simulink model "observateur_terme_integral"  (R2025b)
settings: Solver=FixedStepAuto  StartTime=0.0  StopTime=inf  RelTol=1e-3  EnableMultiTasking=on
values from neighbouring files (symbols this model uses):
  H_barre = K_t(3)    [AncienTest.m]
  K_int = K_t(1:2)    [AncienTest.m]
  Te = 1/100    (= 0.01)    [AncienTest.m]    (also in Test.m)
undefined symbols (not defined in the file or in its folder): Aobs, Bobs, Cobs, Dobs
libraries: legoev3lib x2
settings Model: ExtModeTrigDuration=2  Creator=carol  LastModifiedBy=carol
settings SolverCC: PositivePriorityOrder=on
settings OptimizationCC: DefaultParameterBehavior=Inlined  EnhancedBackFolding=on  PassReuseOutputArgsAs=Individual arguments  ZeroExternalMemoryAtStartup=off  ZeroInternalMemoryAtStartup=off  MaxStackSize=64  OptimizeBlockOrder=speed  DifferentSizesBufferReuse=on  OptimizationCustomize=off  EfficientTunableParamExpr=on
settings DebuggingCC: ParameterTunabilityLossMsg=error
settings HardwareCC: ProdBitPerPointer=32.0  ProdBitPerSizeT=32.0  ProdBitPerPtrDiffT=32.0  ProdLargestAtomicInteger=Long  ProdWordSize=32.0  ProdHWDeviceType=ARM Compatible->ARM 9  UseEmbeddedCoderFeatures=off  UseSimulinkCoderFeatures=off
settings SFSimCC: MATLABDynamicMemAlloc=off
settings RTWCC: SystemTargetFile=ert.tlc  HardwareBoard=LEGO MINDSTORMS EV3  TLCOptions="-aInlineSetEventsForThisBaseRateFcn=TLC_FALSE -aSuppressMultiTaskScheduler=TLC_FALSE  -aRateBasedStepFcn=0"  TemplateMakefile=ert_default_tmf  Toolchain=Sourcery G++ Lite v2009q3  Description=Embedded Coder
settings CodeAppCC: ForceParamTrailComments=on  IgnoreCustomStorageClasses=off  OperatorAnnotations=on  SimulinkDataObjDesc=on  SFDataObjDesc=on  InsertBlockDesc=on
settings ERTTargetCC: ExtModeTransport=2.0  ExtModeStaticAlloc=on  ExtModeMexFile=ext_xcp  ExtModeIntrfLevel=Level2 - Open  SupportContinuousTime=on  SupportNonInlinedSFcns=on  SupportVariableSizeSignals=on

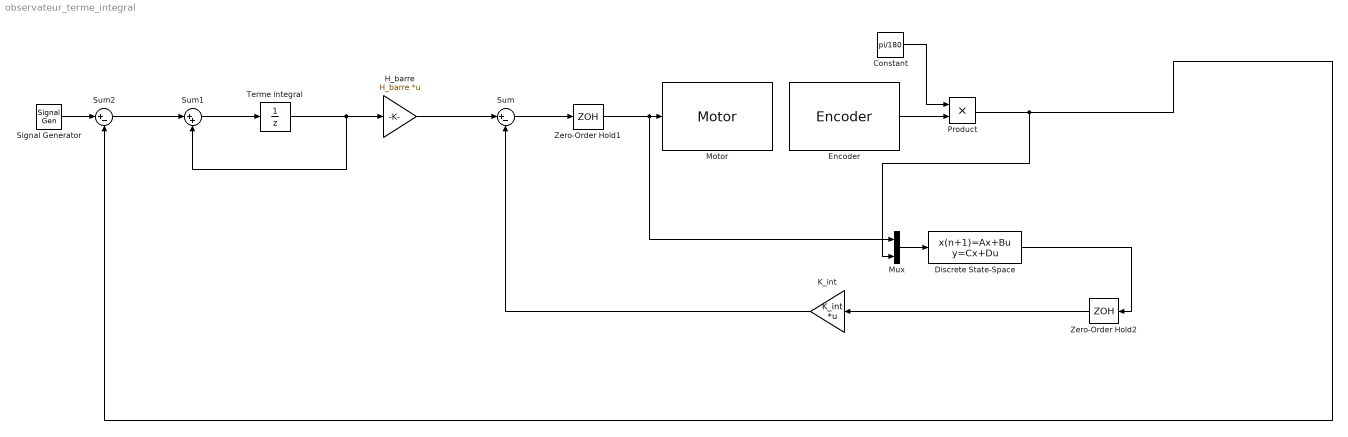
== system observateur_terme_integral ==
  Constant : Constant  Value=pi/180
  Discrete State-Space : DiscreteStateSpace  A=Aobs  B=Bobs  C=Cobs  D=Dobs  SampleTime=Te
  Encoder : legoev3lib/Encoder  portNumber=D  opMode=Reset by external signal  sampleTime=Te
  H_barre : Gain  Gain=H_barre  Multiplication=Matrix(K*u)
  K_int : Gain  Gain=K_int  Multiplication=Matrix(K*u)
  Motor : legoev3lib/Motor  sportNumber=D  sstopAction=Brake
  Mux : Mux  Inputs=2
  Product : Product
  Signal Generator : SignalGenerator  WaveForm=square  Frequency=0.1
  Sum : Sum  Inputs=|+-
  Sum1 : Sum  Inputs=|++
  Sum2 : Sum  Inputs=|+-
  Terme integral : UnitDelay  SampleTime=-1  HasFrameUpgradeWarning=on
  Zero-Order Hold1 : ZeroOrderHold  SampleTime=Te
  Zero-Order Hold2 : ZeroOrderHold  SampleTime=Te
  wires:
  Encoder/1 -> Product/2
  Zero-Order Hold1/1 -> Mux/1, Motor/1
  Sum/1 -> Zero-Order Hold1/1
  H_barre/1 -> Sum/1
  K_int/1 -> Sum/2
  Product/1 -> Mux/2, Sum2/2
  Constant/1 -> Product/1
  Zero-Order Hold2/1 -> K_int/1
  Terme integral/1 -> Sum1/2, H_barre/1
  Sum1/1 -> Terme integral/1
  Sum2/1 -> Sum1/1
  Signal Generator/1 -> Sum2/1
  Mux/1 -> Discrete State-Space/1
  Discrete State-Space/1 -> Zero-Order Hold2/1
